simulink library "simeventssignalmanage1"  (Simulink 7.1)
undefined symbols (not defined in the file or in its folder): des_support, gcbh
libraries: des_sfun_lib x4
settings Model: Creator=Liw  LastModifiedBy=liw  ExtModeAutoUpdateStatusClock=off

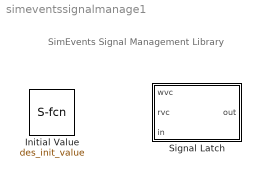
== system simeventssignalmanage1 ==
  note: SimEvents Signal Management Library
  Initial Value : S-Function  LoadFcn=des_support('desSfunLoadFcn',gcbh)  FunctionName=des_init_value  Parameters=InitialValue  EnableBusSupport=off  mask(Initial Value){InitialValue=1}
      mask prompts: InitialValue "Value until first sample time hit:"
      mask help: Output the specified value from the start of the simulation until the first sample time hit at the input port. For the first sample time hit and all subsequent hits, the output signal is identical to the input signal.
      mask init:
      | % For icon display
      | ValueStr = get_param(gcb,'MaskValueString');
      settings: CopyFcn=des_support('desSfunCopyFcn',gcbh)  NameChangeFcn=des_support('desSfunNameChangeFcn',gcbh)
      mask Help: helpview(simeventsbhelp)
      mask Display:
      | image(des_iconLoad('signalInitValue.bmp'),'center')
      | disp([ValueStr '    \n\n'])
  Signal Latch : Subsystem  LoadFcn=des_support('desLoadFcn',gcbh)  StartFcn=des_support('desStartFcn',gcbh)  StopFcn=des_support('desStopFcn',gcbh)  mask(Signal Latch){InitialMemoryValue=0, WriteMemoryUpon=Change in signal from port wvc, MemoryWriteEdgeOption=Rising, SpecifyWriteEventPriority=on, PriorityMemoryWrite=7100, ReadMemoryUpon=Change in signal from port rvc, MemoryReadEdgeOption=Falling, SpecifyReadEventPriority=on, PriorityMemoryRead=7000, ReportMemoryState=off, ReportMemoryUponWrite=off, ReportMemoryUponRead=on}
      mask prompts: InitialMemoryValue "Initial memory value:"; WriteMemoryUpon "Write to memory upon:"; MemoryWriteEdgeOption "Type of change in signal value:"; SpecifyWriteEventPriority "Resolve simultaneous signal updates according to event priority"; PriorityMemoryWrite "Event priority for writing to memory:"; ReadMemoryUpon "Read from memory upon:"; MemoryReadEdgeOption "Type of change in signal value:"; SpecifyReadEventPriority "Resolve simultaneous signal updates according to event priority"; PriorityMemoryRead "Event priority for reading from memory:"; ReportMemoryState "Report state of the block, st"; ReportMemoryUponWrite "Report memory value upon write event, mem"; ReportMemoryUponRead "Report memory value upon read event, out"
      mask help: Write signal value to memory when write to memory event occurs. Read memory value and update out port when read from memory event occurs. The state of the block is 0 if the last event was a read event, and 1 if the last event was a write event.
      mask init:
      | des_sgnlatchmask(gcb, 'init','apply')
      settings: CopyFcn=des_support('desCopyFcn',gcbh)  DeleteFcn=des_support('desDeleteFcn',gcbh)  UndoDeleteFcn=des_support('desUndoDeleteFcn',gcbh)  ModelCloseFcn=des_support('desModelCloseFcn',gcbh)  PreSaveFcn=des_support('desPreSaveFcn',gcbh)  PostSaveFcn=des_support('desPostSaveFcn',gcbh)  NameChangeFcn=des_support('desNameChangeFcn',gcbh)  CloseFcn=des_support('desCloseFcn',gcbh)  ErrorFcn=des_error_redirect
      mask Help: helpview(simeventsbhelp)
      mask StyleString: edit,popup(Sample time hit from port wts|Trigger from port wtr|Change in signal from port wvc|Function call from port wfcn),popup(Rising|Falling|Either),checkbox,edit,popup(Sample time hit from port rts|Trigger from port rtr|Change in signal from port rvc|Function call from port rfcn|Write to memory event),popup(Rising|Falling|Either),checkbox,edit,checkbox,checkbox,checkbox
      mask CallbackString: |des_sgnlatchmask(gcb,'cbWriteMemoryUpon','noapply');||des_sgnlatchmask(gcb,'cbSpecifyWriteEventPriority','noapply');||des_sgnlatchmask(gcb,'cbReadMemoryUpon','noapply');||des_sgnlatchmask(gcb,'cbSpecifyReadEventPriority','noapply');||des_sgnlatchmask(gcb,'cbReportMemoryState','noapply');|des_sgnlatchmask(gcb,'cbReportMemoryUponWrite','noapply');|des_sgnlatchmask(gcb,'cbReportMemoryUponRead','noapply');
      mask TabNameString: Write,Write,Write,Write,Write,Read,Read,Read,Read,Status,Status,Status
      mask Display:
      | image(des_iconLoad('gatesSigLatch.jpg'),'center');
      | port_label('input',1,'wvc');
      | port_label('input',2,'rvc');
      | port_label('input',3,'in');
      | port_label('output',1,'out');

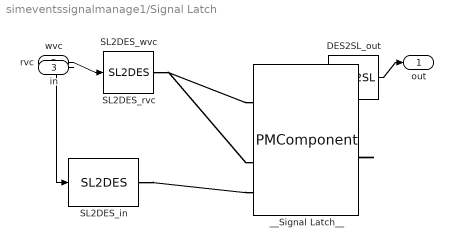
== system simeventssignalmanage1/Signal Latch ==
  wvc : Inport  PortDimensions=1  OutDataTypeStr=double  DataType=double  OutDataType=sfix(16)  OutScaling=2^0
  rvc : Inport  Port=2  PortDimensions=1  OutDataTypeStr=double  DataType=double  OutDataType=sfix(16)  OutScaling=2^0
  in : Inport  Port=3  PortDimensions=1  OutDataTypeStr=double  DataType=double  OutDataType=sfix(16)  OutScaling=2^0
  DES2SL_out : des_sfun_lib/DES2SL  SystemSampleTime=-1  PortType=desPortIn  PhysicalDomain=simevents  SubClassName=DES_DES2SL  timingControl=SimEvents  execIndex=0  multipleOutputs=off  updateBeforeRead=off  InitValue=0  sampleTime=-1  offsetTime=0  idxBlockMR=0  IsMonitorOnly=off  dimsInfo=1
  SL2DES_in : des_sfun_lib/SL2DES  SystemSampleTime=-1  PortType=desPortOut  PhysicalDomain=simevents  SubClassName=DES_SL2DES  timingControl=SimEvents  execIndex=1  trigger=None  filter=0  updateBeforeRead=off  InitValue=0  initToFactVal=off  sampleTime=-1  offsetTime=0  idxBlockMR=0  IsMonitorOnly=off  dimsInfo=1
  SL2DES_rvc : des_sfun_lib/SL2DES  SystemSampleTime=-1  PortType=desPortOut  PhysicalDomain=simevents  SubClassName=DES_SL2DES  timingControl=Simulink  execIndex=7000  trigger=None  filter=0  updateBeforeRead=off  InitValue=0  initToFactVal=off  sampleTime=-1  offsetTime=0  idxBlockMR=0  IsMonitorOnly=off  dimsInfo=1
  SL2DES_wvc : des_sfun_lib/SL2DES  SystemSampleTime=-1  PortType=desPortOut  PhysicalDomain=simevents  SubClassName=DES_SL2DES  timingControl=Simulink  execIndex=7100  trigger=None  filter=0  updateBeforeRead=off  InitValue=0  initToFactVal=off  sampleTime=-1  offsetTime=0  idxBlockMR=0  IsMonitorOnly=off  dimsInfo=1
  __Signal Latch__ : PMComponent  PhysicalDomain=simevents  SubClassName=DES_SIGNAL_LATCH  LeftPortType=desPortIn  RightPortType=desPortOut  LConnTagsString=DI|DI|DI|DI|DI|DI|DI|DI|DI|DI  RConnTagsString=DO|DO|DO|DO
      mask Display:
      | port_label('LConn',1,'wts');
      | port_label('LConn',2,'wtr');
      | port_label('LConn',3,'wvc');
      | port_label('LConn',4,'wfcn');
      | port_label('LConn',5,'rts');
      | port_label('LConn',6,'rtr');
      | port_label('LConn',7,'rvc');
      | port_label('LConn',8,'rfcn');
      | port_label('LConn',9,'in');
      | port_label('LConn',10,'IN');
      | port_label('RConn',1,'st');
      | port_label('RConn',2,'mem');
      | port_label('RConn',3,'out');
      | port_label('RConn',4,'OUT');
  out : Outport  OutDataTypeStr=double  DataType=double  OutDataType=sfix(16)  OutScaling=2^0
  wires:
  rvc/1 -> SL2DES_rvc/1
  wvc/1 -> SL2DES_wvc/1
  in/1 -> SL2DES_in/1
  DES2SL_out/1 -> out/1
  connections:
  SL2DES_rvc/RConn1 -- __Signal Latch__/LConn7
  SL2DES_wvc/RConn1 -- __Signal Latch__/LConn3
  SL2DES_in/RConn1 -- __Signal Latch__/LConn9
  __Signal Latch__/RConn3 -- DES2SL_out/LConn1
